simulink model "FDIBenchMark_66"  (Simulink 7.0)
settings: Solver=ode45  StartTime=0.0  StopTime=4400  FixedStep=Ts  RelTol=1e-12
InitFcn:
  | FDIBenchMarkData
values from neighbouring files (symbols this model uses):
  a = 2.2    [FDIBenchMarkData.m]
  Addt = [-(B_dt+B_r)/J_r B_dt/N_g/J_r -K_dt/J_r; eta_dt*B_dt/N_g/J_g -(eta_dt*B_dt/N_g^2+B_g)/J_g eta_dt*K_dt/N_g/J_g; 1 -1/N_g 0]    [FDIBenchMarkData.m]
  Addt2 = [-(B_dt+B_r)/J_r B_dt/N_g/J_r -K_dt/J_r; eta_dt2*B_dt/N_g/J_g -(eta_dt2*B_dt/N_g^2+B_g)/J_g eta_dt2*K_dt/N_g/J_g; 1 -1/N_g 0]    [FDIBenchMarkData.m]
  alpha = 0.1    [FDIBenchMarkData.m]
  alpha_gc = 50    [FDIBenchMarkData.m]
  Bddt = [1/J_r 0; 0 -1/J_g;0 0]    [FDIBenchMarkData.m]
  Bddt2 = [1/J_r 0; 0 -1/J_g;0 0]    [FDIBenchMarkData.m]
  Cddt = [1 0 0;0 1 0]    [FDIBenchMarkData.m]
  Constant_Beta_1_m1 = 5    [FDIBenchMarkData.m]
  Constant_Beta_3_m1 = 10    [FDIBenchMarkData.m]
  Constant_Omega_r_m1 = 1.4    [FDIBenchMarkData.m]
  Constant_tau_gc = 100    [FDIBenchMarkData.m]
  eta_gc = 0.98    [FDIBenchMarkData.m]
  Gain_Beta_2_m2 = 1.2    [FDIBenchMarkData.m]
  Gain_Omega_r_m2 = 1.1    [FDIBenchMarkData.m]
  H = 87    [FDIBenchMarkData.m]
  k = 4.7    [FDIBenchMarkData.m]
  K_i = 1    [FDIBenchMarkData.m]
  K_opt = .5* rho* pi*R^2*eta_dt*R^3*0.4554/(N_g*8)^3    (= 1.21708013189)    [FDIBenchMarkData.m]
  K_p = 4    [FDIBenchMarkData.m]
  L = acker(A', C', vpe)'    [FDIBenchMarkData.m]
  m = 1+alpha*(alpha-1)*R^2/(8*H^2)    (= 0.995085835315)    [FDIBenchMarkData.m]
  m_Beta = 0    [FDIBenchMarkData.m]
  m_omega_g = 0    [FDIBenchMarkData.m]
  m_omega_r = 0    [FDIBenchMarkData.m]
  m_P_g = 0    [FDIBenchMarkData.m]
  m_tau_g = 0    [FDIBenchMarkData.m]
  m_vw = 1.5    [FDIBenchMarkData.m]
  Omega_delta = 15    [FDIBenchMarkData.m]
  omega_n = 11.11    [FDIBenchMarkData.m]
  Omega_nom = 162    [FDIBenchMarkData.m]
  P_r = 4.8e6    (= 4800000)    [FDIBenchMarkData.m]
  R = 57.5    [FDIBenchMarkData.m]
  r = D_rotor/2    (= 57.5)    [FDIBenchMarkData.m]
  r0 = 1.5    [FDIBenchMarkData.m]
  rho = 1.225    [FDIBenchMarkData.m]
  seed = ceil(seed)    [FDIBenchMarkData.m]
  sigma_Beta = 0.2    [FDIBenchMarkData.m]
  sigma_omega_g = 0.05    [FDIBenchMarkData.m]
  sigma_omega_r = 0.004*2*pi    (= 0.0251327412287)    [FDIBenchMarkData.m]
  sigma_P_g = 1e3    (= 1000)    [FDIBenchMarkData.m]
  sigma_tau_g = 90    [FDIBenchMarkData.m]
  sigma_vm = 0.5    [FDIBenchMarkData.m]
  T_sample = 0.05    [FDIBenchMarkData.m]
  Ts = 1/100    (= 0.01)    [FDIBenchMarkData.m]
  turb_int = Turbulence_intensity    (= 12)    [FDIBenchMarkData.m]
  turbulence_seeds = [seed1 seed2]    [FDIBenchMarkData.m]
  xi = 0.6    [FDIBenchMarkData.m]
undefined symbols (not defined in the file or in its folder): Apb, Apb1, Apb2, Bpb, Bpb1, Bpb2, Cpb, Cpb1, Cpb2, Cq, DiscIntNeverNeededParam, u0
(part 1 of 2)
settings Model: Creator=peodg  LastModifiedBy=peodg
settings SolverCC: MaxConsecutiveZCs=1e6
settings HardwareCC: TargetHWDeviceType=32-bit Generic
settings GRTTargetCC: TargetFcnLib=ansi_tfl_tmw.mat

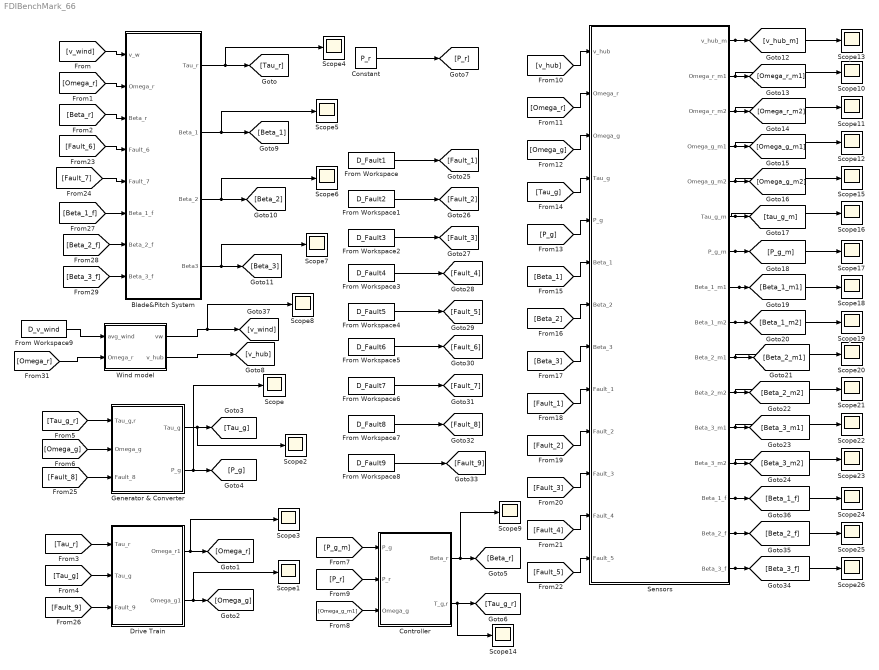
== system FDIBenchMark_66 ==
  Blade&Pitch System : Subsystem
  Constant : Constant  Value=P_r  OutDataType=sfix(16)  OutScaling=2^0
  Controller : Subsystem
  Drive Train : Subsystem
  From Workspace : FromWorkspace  VariableName=D_Fault1  SampleTime=Ts
  From Workspace1 : FromWorkspace  VariableName=D_Fault2  SampleTime=Ts
  From Workspace2 : FromWorkspace  VariableName=D_Fault3  SampleTime=Ts
  From Workspace3 : FromWorkspace  VariableName=D_Fault4  SampleTime=Ts
  From Workspace4 : FromWorkspace  VariableName=D_Fault5  SampleTime=Ts
  From Workspace5 : FromWorkspace  VariableName=D_Fault6  SampleTime=Ts
  From Workspace6 : FromWorkspace  VariableName=D_Fault7  SampleTime=Ts
  From Workspace7 : FromWorkspace  VariableName=D_Fault8  SampleTime=Ts
  From Workspace8 : FromWorkspace  VariableName=D_Fault9  SampleTime=Ts
  From Workspace9 : FromWorkspace  VariableName=D_v_wind
  Generator & Converter : Subsystem
  Scope{,1..26} (27 alike) : Scope
      Scope settings: YMin=1e+006  YMax=5.25e+006  SaveName=P_g  DataFormat=Array  SampleInput=on  SampleTime=Ts
      Scope1 settings: YMin=64  YMax=66.25  SaveName=Oemga_g1  DataFormat=Array  SampleInput=on  SampleTime=Ts
      Scope10 settings: YMin=1.1  YMax=2.4  SaveName=Omega_r_m1  DataFormat=Array  SampleInput=on  SampleTime=Ts
      Scope11 settings: YMin=-1  YMax=1  SaveName=Omega_r_m2  DataFormat=Array  SampleInput=on  SampleTime=Ts
      Scope12 settings: YMin=-1  YMax=1  SaveName=Omega_g_m1  DataFormat=Array  SampleInput=on  SampleTime=Ts
      Scope13 settings: YMin=-1  YMax=1  SaveName=v_hub_m  DataFormat=Array  SampleInput=on  SampleTime=Ts
      Scope14 settings: YMin=-2.5  YMax=20  SaveName=T_g_r  DataFormat=Array  SampleInput=on  SampleTime=Ts
      Scope15 settings: YMin=-1  YMax=1  SaveName=Omega_g_m2  DataFormat=Array  SampleInput=on  SampleTime=Ts
      Scope16 settings: YMin=-1  YMax=1  SaveName=Tau_g_m  DataFormat=Array  SampleInput=on  SampleTime=Ts
      Scope17 settings: YMin=-1  YMax=1  SaveName=P_g_m  DataFormat=Array  SampleInput=on  SampleTime=Ts
      Scope18 settings: YMin=-1  YMax=1  SaveName=Beta_1_m1  DataFormat=Array  SampleInput=on  SampleTime=Ts
      Scope19 settings: YMin=-1  YMax=1  SaveName=Beta_1_m2  DataFormat=Array  SampleInput=on  SampleTime=Ts
      Scope2 settings: YMin=29400  YMax=29875  SaveName=Tau_g  DataFormat=Array  SampleInput=on  SampleTime=Ts
      Scope20 settings: YMin=-1  YMax=1  SaveName=Beta_2_m1  DataFormat=Array  SampleInput=on  SampleTime=Ts
      Scope21 settings: YMin=-1  YMax=1  SaveName=Beta_2_m2  DataFormat=Array  SampleInput=on  SampleTime=Ts
      Scope22 settings: YMin=-1  YMax=1  SaveName=Beta_3_m1  DataFormat=Array  SampleInput=on  SampleTime=Ts
      Scope23 settings: YMin=-1  YMax=1  SaveName=Beta_3_m2  DataFormat=Array  SampleInput=on  SampleTime=Ts
      Scope24 settings: YMin=-1  YMax=1  SaveName=Beta_1_f  DataFormat=Array  SampleInput=on  SampleTime=Ts
      Scope25 settings: YMin=-1  YMax=1  SaveName=Beta_2_f  DataFormat=Array  SampleInput=on  SampleTime=Ts
      Scope26 settings: YMin=-1  YMax=1  SaveName=Beta_3_f  DataFormat=Array  SampleInput=on  SampleTime=Ts
      Scope3 settings: YMin=0.62  YMax=0.69  SaveName=Omega_r1  DataFormat=Array  SampleInput=on  SampleTime=Ts
      Scope4 settings: YMin=-1e+006  YMax=6e+006  SaveName=Tau_r  DataFormat=Array  SampleInput=on  SampleTime=Ts
      Scope5 settings: YMin=-3  YMax=8  SaveName=Beta1  DataFormat=Array  SampleInput=on  SampleTime=Ts
      Scope6 settings: YMin=-0.3  YMax=0.3  SaveName=Beta  DataFormat=Array  SampleInput=on  SampleTime=Ts
      Scope7 settings: YMin=-0.25  YMax=0.35  SaveName=Beta3  DataFormat=Array  SampleInput=on  SampleTime=Ts
      Scope8 settings: YMin=3  YMax=18  SaveName=Vw  DataFormat=Array  SampleInput=on  SampleTime=Ts
      Scope9 settings: YMin=-2.5  YMax=20  SaveName=Beta_r  DataFormat=Array  SampleInput=on  SampleTime=Ts
  Sensors : Subsystem
  Wind model : Subsystem
  wires:
  [v_wind] -> Blade&Pitch System/1(v_w)
  [Omega_r] -> Blade&Pitch System/2(Omega_r)
  [Beta_r] -> Blade&Pitch System/3(Beta_r)
  [Tau_r] -> Drive Train/1(Tau_r)
  [Tau_g] -> Drive Train/2(Tau_g)
  Drive Train/1(Omega_r1) -> [Omega_r], Scope3/1
  [Tau_g_r] -> Generator & Converter/1(Tau_g,r)
  [Omega_g] -> Generator & Converter/2(Omega_g)
  Generator & Converter/1(Tau_g) -> [Tau_g], Scope2/1
  Generator & Converter/2(P_g) -> [P_g], Scope/1
  [P_g_m] -> Controller/1(P_g)
  [Omega_g_m1] -> Controller/3(Omega_g)
  Controller/1(Beta_r) -> [Beta_r], Scope9/1
  Controller/2(T_g,r) -> [Tau_g_r], Scope14/1
  [P_r] -> Controller/2(P_r)
  Constant/1 -> [P_r]
  Sensors/1(v_hub_m) -> [v_hub_m], Scope13/1
  Sensors/2(Omega_r_m1) -> [Omega_r_m1], Scope10/1
  Sensors/3(Omega_r_m2) -> [Omega_r_m2], Scope11/1
  Sensors/4(Omega_g_m1) -> [Omega_g_m1], Scope12/1
  Sensors/5(Omega_g_m2) -> [Omega_g_m2], Scope15/1
  Sensors/6(Tau_g_m) -> [tau_g_m], Scope16/1
  Sensors/7(P_g_m) -> [P_g_m], Scope17/1
  Sensors/8(Beta_1_m1) -> [Beta_1_m1], Scope18/1
  Sensors/9(Beta_1_m2) -> [Beta_1_m2], Scope19/1
  Sensors/10(Beta_2_m1) -> [Beta_2_m1], Scope20/1
  Sensors/11(Beta_2_m2) -> [Beta_2_m2], Scope21/1
  Sensors/12(Beta_3_m1) -> [Beta_3_m1], Scope22/1
  Sensors/13(Beta_3_m2) -> [Beta_3_m2], Scope23/1
  [v_hub] -> Sensors/1(v_hub)
  [Omega_r] -> Sensors/2(Omega_r)
  [Omega_g] -> Sensors/3(Omega_g)
  [Tau_g] -> Sensors/4(Tau_g)
  [P_g] -> Sensors/5(P_g)
  [Beta_1] -> Sensors/6(Beta_1)
  [Beta_2] -> Sensors/7(Beta_2)
  [Beta_3] -> Sensors/8(Beta_3)
  [Fault_1] -> Sensors/9(Fault_1)
  [Fault_2] -> Sensors/10(Fault_2)
  [Fault_3] -> Sensors/11(Fault_3)
  [Fault_4] -> Sensors/12(Fault_4)
  [Fault_5] -> Sensors/13(Fault_5)
  [Fault_6] -> Blade&Pitch System/4(Fault_6)
  [Fault_7] -> Blade&Pitch System/5(Fault_7)
  [Fault_8] -> Generator & Converter/3(Fault_8)
  [Fault_9] -> Drive Train/3(Fault_9)
  From Workspace8/1 -> [Fault_9]
  From Workspace7/1 -> [Fault_8]
  From Workspace6/1 -> [Fault_7]
  From Workspace5/1 -> [Fault_6]
  From Workspace4/1 -> [Fault_5]
  From Workspace3/1 -> [Fault_4]
  From Workspace2/1 -> [Fault_3]
  From Workspace1/1 -> [Fault_2]
  From Workspace/1 -> [Fault_1]
  Drive Train/2(Omega_g1) -> [Omega_g], Scope1/1
  Sensors/16(Beta_3_f) -> [Beta_3_f], Scope26/1
  Sensors/15(Beta_2_f) -> [Beta_2_f], Scope25/1
  Sensors/14(Beta_1_f) -> [Beta_1_f], Scope24/1
  [Beta_1_f] -> Blade&Pitch System/6(Beta_1_f)
  [Beta_2_f] -> Blade&Pitch System/7(Beta_2_f)
  [Beta_3_f] -> Blade&Pitch System/8(Beta_3_f)
  Blade&Pitch System/4(Beta3) -> [Beta_3], Scope7/1
  Blade&Pitch System/3(Beta_2) -> [Beta_2], Scope6/1
  Blade&Pitch System/2(Beta_1) -> [Beta_1], Scope5/1
  Blade&Pitch System/1(Tau_r) -> [Tau_r], Scope4/1
  Wind model/1(vw) -> [v_wind], Scope8/1
  Wind model/2(v_hub) -> [v_hub]
  [Omega_r] -> Wind model/2(Omega_r)
  From Workspace9/1 -> Wind model/1(avg_wind)

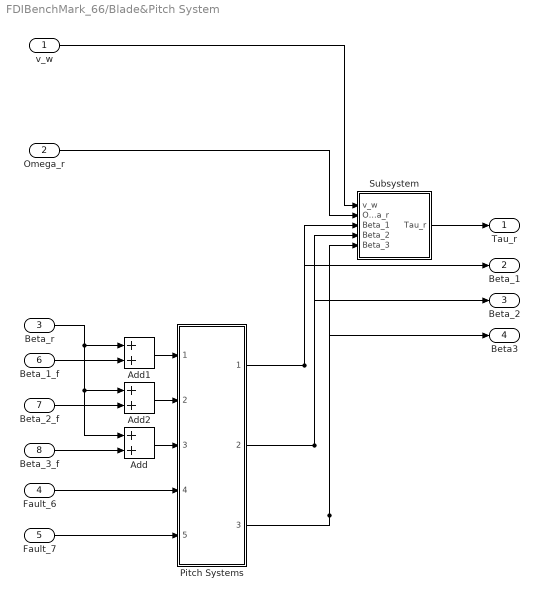
== system FDIBenchMark_66/Blade&Pitch System ==
  v_w : Inport  OutDataType=sfix(16)  OutScaling=2^0
  Omega_r : Inport  Port=2  OutDataType=sfix(16)  OutScaling=2^0
  Beta_r : Inport  Port=3  OutDataType=sfix(16)  OutScaling=2^0
  Fault_6 : Inport  Port=4  OutDataType=sfix(16)  OutScaling=2^0
  Fault_7 : Inport  Port=5  OutDataType=sfix(16)  OutScaling=2^0
  Beta_1_f : Inport  Port=6  OutDataType=sfix(16)  OutScaling=2^0
  Beta_2_f : Inport  Port=7  OutDataType=sfix(16)  OutScaling=2^0
  Beta_3_f : Inport  Port=8  OutDataType=sfix(16)  OutScaling=2^0
  Add : Sum  OutDataType=sfix(16)  OutScaling=2^-10
  Add1 : Sum  OutDataType=sfix(16)  OutScaling=2^-10
  Add2 : Sum  OutDataType=sfix(16)  OutScaling=2^-10
  Pitch Systems : Subsystem
  Subsystem : Subsystem
  Tau_r : Outport  OutDataType=sfix(16)  OutScaling=2^0
  Beta_1 : Outport  Port=2  OutDataType=sfix(16)  OutScaling=2^0
  Beta_2 : Outport  Port=3  OutDataType=sfix(16)  OutScaling=2^0
  Beta3 : Outport  Port=4  OutDataType=sfix(16)  OutScaling=2^0
  wires:
  Pitch Systems/1(Beta_1) -> Subsystem/3(Beta_1), Beta_1/1
  Pitch Systems/2(Beta_2) -> Subsystem/4(Beta_2), Beta_2/1
  Pitch Systems/3(Beta_3) -> Subsystem/5(Beta_3), Beta3/1
  Subsystem/1(Tau_r) -> Tau_r/1
  v_w/1 -> Subsystem/1(v_w)
  Omega_r/1 -> Subsystem/2(Omega_r)
  Fault_6/1 -> Pitch Systems/4(Fault_6)
  Fault_7/1 -> Pitch Systems/5(Fault_7)
  Add/1 -> Pitch Systems/3(Beta_r3)
  Add1/1 -> Pitch Systems/1(Beta_r1)
  Add2/1 -> Pitch Systems/2(Beta_r2)
  Beta_3_f/1 -> Add/2
  Beta_2_f/1 -> Add2/2
  Beta_1_f/1 -> Add1/2
  Beta_r/1 -> Add1/1, Add2/1, Add/1

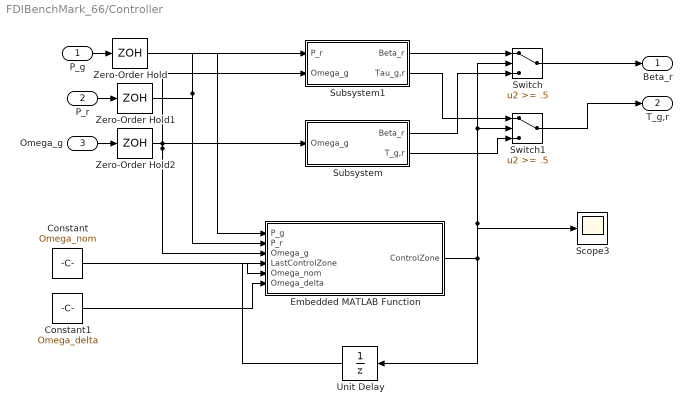
== system FDIBenchMark_66/Controller ==
  P_g : Inport  OutDataType=sfix(16)  OutScaling=2^0
  P_r : Inport  Port=2  OutDataType=sfix(16)  OutScaling=2^0
  Omega_g : Inport  Port=3  OutDataType=sfix(16)  OutScaling=2^0
  Constant : Constant  Value=Omega_nom  OutDataType=sfix(16)  OutScaling=2^0
  Constant1 : Constant  Value=Omega_delta  OutDataType=sfix(16)  OutScaling=2^0
  Embedded MATLAB Function : Stateflow chart
      settings: PermitHierarchicalResolution=ParametersOnly
  Scope3 : Scope
      settings: YMin=0.62  YMax=0.69  SaveName=Omega_r  DataFormat=Array  SampleInput=on  SampleTime=Ts
  Subsystem : Subsystem
  Subsystem1 : Subsystem
  Switch : Switch  Threshold=.5
  Switch1 : Switch  Threshold=.5
  Unit Delay : UnitDelay  Orientation=left  SampleTime=Ts
  Zero-Order Hold : ZeroOrderHold  SampleTime=Ts
  Zero-Order Hold1 : ZeroOrderHold  SampleTime=Ts
  Zero-Order Hold2 : ZeroOrderHold  SampleTime=Ts
  Beta_r : Outport  OutDataType=sfix(16)  OutScaling=2^0
  T_g,r : Outport  Port=2  OutDataType=sfix(16)  OutScaling=2^0
  wires:
  Embedded MATLAB Function/1(ControlZone) -> Unit Delay/1, Switch/2, Switch1/2, Scope3/1
  Unit Delay/1 -> Embedded MATLAB Function/4(LastControlZone)
  P_g/1 -> Zero-Order Hold/1
  P_r/1 -> Zero-Order Hold1/1
  Omega_g/1 -> Zero-Order Hold2/1
  Switch/1 -> Beta_r/1
  Switch1/1 -> T_g,r/1
  Subsystem1/1(Beta_r) -> Switch/1
  Subsystem/1(Beta_r) -> Switch/3
  Subsystem1/2(Tau_g,r) -> Switch1/1
  Subsystem/2(T_g,r) -> Switch1/3
  Constant/1 -> Embedded MATLAB Function/5(Omega_nom)
  Constant1/1 -> Embedded MATLAB Function/6(Omega_delta)
  Zero-Order Hold/1 -> Embedded MATLAB Function/1(P_g)
  Zero-Order Hold1/1 -> Embedded MATLAB Function/2(P_r), Subsystem1/1(P_r)
  Zero-Order Hold2/1 -> Embedded MATLAB Function/3(Omega_g), Subsystem1/2(Omega_g), Subsystem/1(Omega_g)

== system FDIBenchMark_66/Drive Train ==
  Tau_r : Inport  OutDataType=sfix(16)  OutScaling=2^0
  Tau_g : Inport  Port=2  OutDataType=sfix(16)  OutScaling=2^0
  Fault_9 : Inport  Port=3  OutDataType=sfix(16)  OutScaling=2^0
  Add : Sum  OutDataType=sfix(16)  OutScaling=2^-10
  Demux1 : Demux  Outputs=2
  Gain : Gain  Orientation=left  Gain=Addt  Multiplication=Matrix(K*u)  ParameterDataType=sfix(16)  ParameterScaling=2^0  OutDataType=sfix(16)  OutScaling=2^0
  Gain1 : Gain  Gain=Bddt  Multiplication=Matrix(K*u)  ParameterDataType=sfix(16)  ParameterScaling=2^0  OutDataType=sfix(16)  OutScaling=2^0
  Gain2 : Gain  Gain=Cddt  Multiplication=Matrix(K*u)  ParameterDataType=sfix(16)  ParameterScaling=2^0  OutDataType=sfix(16)  OutScaling=2^0
  Gain3 : Gain  Orientation=left  Gain=Addt2  Multiplication=Matrix(K*u)  ParameterDataType=sfix(16)  ParameterScaling=2^0  OutDataType=sfix(16)  OutScaling=2^0
  Gain4 : Gain  Gain=Bddt2  Multiplication=Matrix(K*u)  ParameterDataType=sfix(16)  ParameterScaling=2^0  OutDataType=sfix(16)  OutScaling=2^0
  Integrator : Integrator  InitialCondition=[1 100 0]
  Mux : Mux  Inputs=2
  Switch1 : Switch  Threshold=0.5
  Switch2 : Switch  Orientation=left  Threshold=0.5
  Omega_r1 : Outport  OutDataType=sfix(16)  OutScaling=2^0
  Omega_g1 : Outport  Port=2  OutDataType=sfix(16)  OutScaling=2^0
  wires:
  Tau_r/1 -> Mux/1
  Tau_g/1 -> Mux/2
  Integrator/1 -> Gain2/1, Gain/1, Gain3/1
  Add/1 -> Integrator/1
  Switch1/1 -> Add/1
  Gain1/1 -> Switch1/1
  Gain4/1 -> Switch1/3
  Gain/1 -> Switch2/1
  Gain3/1 -> Switch2/3
  Switch2/1 -> Add/2
  Demux1/1 -> Omega_r1/1
  Demux1/2 -> Omega_g1/1
  Gain2/1 -> Demux1/1
  Fault_9/1 -> Switch1/2, Switch2/2
  Mux/1 -> Gain1/1, Gain4/1

== system FDIBenchMark_66/Generator & Converter ==
  Tau_g,r : Inport  OutDataType=sfix(16)  OutScaling=2^0
  Omega_g : Inport  Port=2  OutDataType=sfix(16)  OutScaling=2^0
  Fault_8 : Inport  Port=3  OutDataType=sfix(16)  OutScaling=2^0
  Bias : Bias  Bias=Constant_tau_gc
  Divide : Product  Inputs=**  OutDataType=sfix(16)  OutScaling=2^-10
  Gain : Gain  Gain=eta_gc  ParameterDataType=sfix(16)  ParameterScaling=2^0  OutDataType=sfix(16)  OutScaling=2^0
  Switch : Switch  Threshold=0.5
  Transfer Fcn : TransferFcn  Numerator=[alpha_gc]  Denominator=[1 alpha_gc]
  Tau_g : Outport  OutDataType=sfix(16)  OutScaling=2^0
  P_g : Outport  Port=2  OutDataType=sfix(16)  OutScaling=2^0
  wires:
  Tau_g,r/1 -> Transfer Fcn/1
  Gain/1 -> P_g/1
  Divide/1 -> Gain/1
  Omega_g/1 -> Divide/2
  Transfer Fcn/1 -> Bias/1, Switch/1
  Fault_8/1 -> Switch/2
  Switch/1 -> Divide/1, Tau_g/1
  Bias/1 -> Switch/3

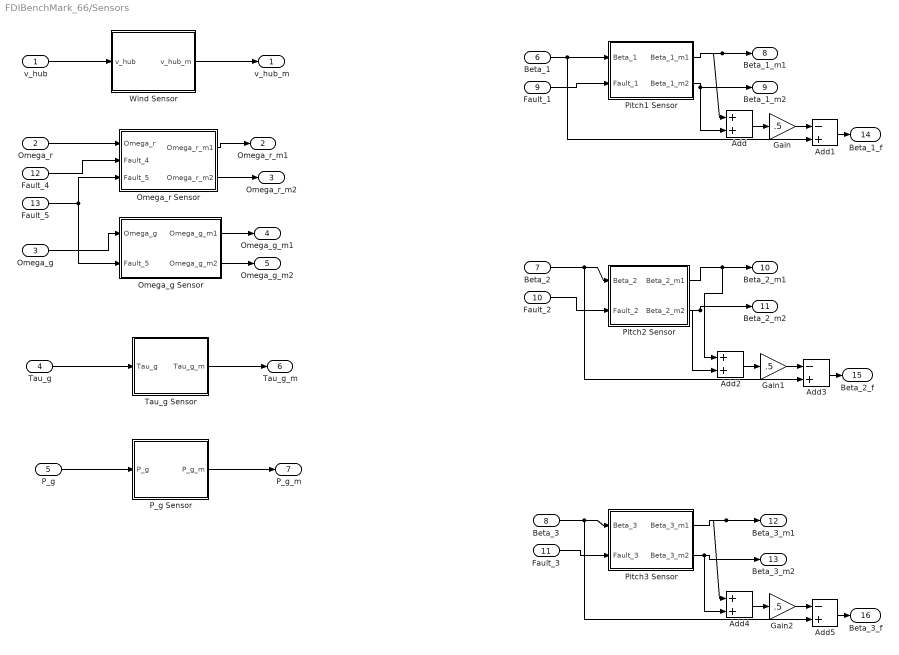
== system FDIBenchMark_66/Sensors ==
  v_hub : Inport  OutDataType=sfix(16)  OutScaling=2^0
  Omega_r : Inport  Port=2  OutDataType=sfix(16)  OutScaling=2^0
  Omega_g : Inport  Port=3  OutDataType=sfix(16)  OutScaling=2^0
  Tau_g : Inport  Port=4  OutDataType=sfix(16)  OutScaling=2^0
  P_g : Inport  Port=5  OutDataType=sfix(16)  OutScaling=2^0
  Beta_1 : Inport  Port=6  OutDataType=sfix(16)  OutScaling=2^0
  Beta_2 : Inport  Port=7  OutDataType=sfix(16)  OutScaling=2^0
  Beta_3 : Inport  Port=8  OutDataType=sfix(16)  OutScaling=2^0
  Fault_1 : Inport  Port=9  OutDataType=sfix(16)  OutScaling=2^0
  Fault_2 : Inport  Port=10  OutDataType=sfix(16)  OutScaling=2^0
  Fault_3 : Inport  Port=11  OutDataType=sfix(16)  OutScaling=2^0
  Fault_4 : Inport  Port=12  OutDataType=sfix(16)  OutScaling=2^0
  Fault_5 : Inport  Port=13  OutDataType=sfix(16)  OutScaling=2^0
  Add : Sum  OutDataType=sfix(16)  OutScaling=2^-10
  Add1 : Sum  Inputs=-+  OutDataType=sfix(16)  OutScaling=2^-10
  Add2 : Sum  OutDataType=sfix(16)  OutScaling=2^-10
  Add3 : Sum  Inputs=-+  OutDataType=sfix(16)  OutScaling=2^-10
  Add4 : Sum  OutDataType=sfix(16)  OutScaling=2^-10
  Add5 : Sum  Inputs=-+  OutDataType=sfix(16)  OutScaling=2^-10
  Gain : Gain  Gain=.5  ParameterDataType=sfix(16)  ParameterScaling=2^0  OutDataType=sfix(16)  OutScaling=2^0
  Gain1 : Gain  Gain=.5  ParameterDataType=sfix(16)  ParameterScaling=2^0  OutDataType=sfix(16)  OutScaling=2^0
  Gain2 : Gain  Gain=.5  ParameterDataType=sfix(16)  ParameterScaling=2^0  OutDataType=sfix(16)  OutScaling=2^0
  Omega_g Sensor : Subsystem
  Omega_r Sensor : Subsystem
  P_g Sensor : Subsystem
  Pitch1 Sensor : Subsystem
  Pitch2 Sensor : Subsystem
  Pitch3 Sensor : Subsystem
  Tau_g Sensor : Subsystem
  Wind Sensor : Subsystem
  v_hub_m : Outport  OutDataType=sfix(16)  OutScaling=2^0
  Omega_r_m1 : Outport  Port=2  OutDataType=sfix(16)  OutScaling=2^0
  Omega_r_m2 : Outport  Port=3  OutDataType=sfix(16)  OutScaling=2^0
  Omega_g_m1 : Outport  Port=4  OutDataType=sfix(16)  OutScaling=2^0
  Omega_g_m2 : Outport  Port=5  OutDataType=sfix(16)  OutScaling=2^0
  Tau_g_m : Outport  Port=6  OutDataType=sfix(16)  OutScaling=2^0
  P_g_m : Outport  Port=7  OutDataType=sfix(16)  OutScaling=2^0
  Beta_1_m1 : Outport  Port=8  OutDataType=sfix(16)  OutScaling=2^0
  Beta_1_m2 : Outport  Port=9  OutDataType=sfix(16)  OutScaling=2^0
  Beta_2_m1 : Outport  Port=10  OutDataType=sfix(16)  OutScaling=2^0
  Beta_2_m2 : Outport  Port=11  OutDataType=sfix(16)  OutScaling=2^0
  Beta_3_m1 : Outport  Port=12  OutDataType=sfix(16)  OutScaling=2^0
  Beta_3_m2 : Outport  Port=13  OutDataType=sfix(16)  OutScaling=2^0
  Beta_1_f : Outport  Port=14  OutDataType=sfix(16)  OutScaling=2^0
  Beta_2_f : Outport  Port=15  OutDataType=sfix(16)  OutScaling=2^0
  Beta_3_f : Outport  Port=16  OutDataType=sfix(16)  OutScaling=2^0
  wires:
  Wind Sensor/1(v_hub_m) -> v_hub_m/1
  v_hub/1 -> Wind Sensor/1(v_hub)
  Omega_r/1 -> Omega_r Sensor/1(Omega_r)
  Omega_r Sensor/1(Omega_r_m1) -> Omega_r_m1/1
  Omega_r Sensor/2(Omega_r_m2) -> Omega_r_m2/1
  Omega_g/1 -> Omega_g Sensor/1(Omega_g)
  Omega_g Sensor/1(Omega_g_m1) -> Omega_g_m1/1
  Omega_g Sensor/2(Omega_g_m2) -> Omega_g_m2/1
  Tau_g/1 -> Tau_g Sensor/1(Tau_g)
  Tau_g Sensor/1(Tau_g_m) -> Tau_g_m/1
  P_g/1 -> P_g Sensor/1(P_g)
  P_g Sensor/1(P_g_m) -> P_g_m/1
  Beta_1/1 -> Pitch1 Sensor/1(Beta_1), Add1/2
  Pitch1 Sensor/1(Beta_1_m1) -> Beta_1_m1/1, Add/1
  Pitch1 Sensor/2(Beta_1_m2) -> Beta_1_m2/1, Add/2
  Beta_2/1 -> Pitch2 Sensor/1(Beta_2), Add3/2
  Pitch2 Sensor/1(Beta_2_m1) -> Beta_2_m1/1, Add2/1
  Pitch2 Sensor/2(Beta_2_m2) -> Beta_2_m2/1, Add2/2
  Beta_3/1 -> Pitch3 Sensor/1(Beta_3), Add5/2
  Pitch3 Sensor/1(Beta_3_m1) -> Beta_3_m1/1, Add4/1
  Pitch3 Sensor/2(Beta_3_m2) -> Beta_3_m2/1, Add4/2
  Fault_1/1 -> Pitch1 Sensor/2(Fault_1)
  Fault_2/1 -> Pitch2 Sensor/2(Fault_2)
  Fault_3/1 -> Pitch3 Sensor/2(Fault_3)
  Fault_4/1 -> Omega_r Sensor/2(Fault_4)
  Fault_5/1 -> Omega_r Sensor/3(Fault_5), Omega_g Sensor/2(Fault_5)
  Add/1 -> Gain/1
  Gain/1 -> Add1/1
  Add1/1 -> Beta_1_f/1
  Add2/1 -> Gain1/1
  Gain1/1 -> Add3/1
  Add3/1 -> Beta_2_f/1
  Add4/1 -> Gain2/1
  Gain2/1 -> Add5/1
  Add5/1 -> Beta_3_f/1

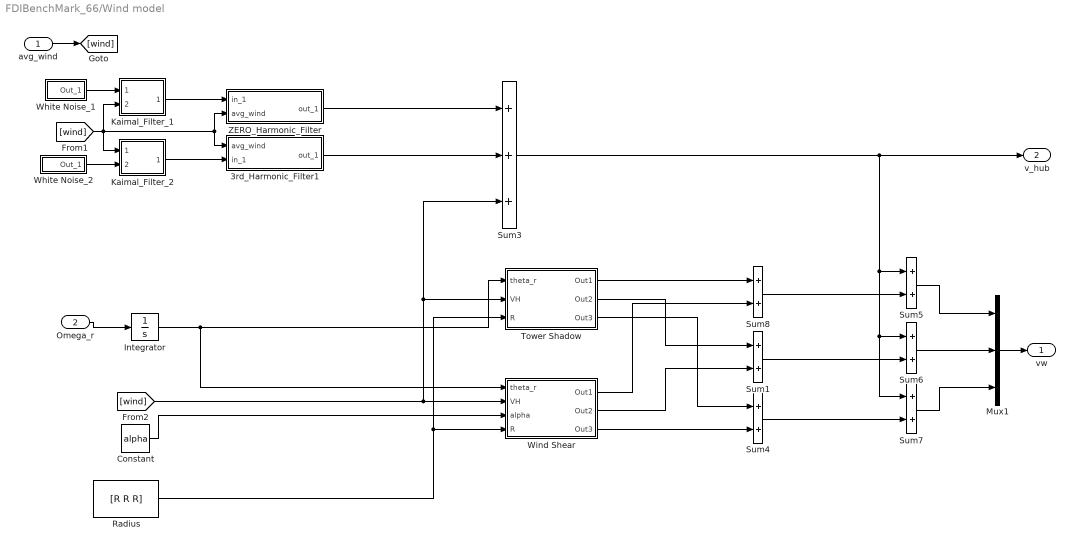
== system FDIBenchMark_66/Wind model ==
  avg_wind : Inport  OutDataType=sfix(16)  OutScaling=2^0
  Omega_r : Inport  Port=2  OutDataType=sfix(16)  OutScaling=2^0
  3rd_Harmonic_Filter1 : Subsystem
  Constant : Constant  Value=alpha  OutDataType=sfix(16)  OutScaling=2^0
  Integrator : Integrator
  Kaimal_Filter_1 : Subsystem
  Kaimal_Filter_2 : Subsystem
  Mux1 : Mux  Inputs=3
  Radius : Constant  Value=[R R R]  OutDataType=sfix(16)  OutScaling=2^0
  Sum{1,4..8} (6 alike) : Sum  OutDataType=sfix(16)  OutScaling=2^0  SaturateOnIntegerOverflow=on  InputSameDT=on
  Sum3 : Sum  Inputs=+++  OutDataType=sfix(16)  OutScaling=2^0  SaturateOnIntegerOverflow=on  InputSameDT=on
  Tower Shadow : Subsystem
  White Noise_1 : Subsystem  mask(Continuous White Noise.){Cov=[1], Ts=T_sample, seed=turbulence_seeds(1)}
      mask prompts: Cov "Noise Power:"; Ts "Sample Time:"
      mask help:
      | White noise for continuous (s-domain) systems.
      | Band-limited using zero-order-hold.
      mask init:
      | r = rand(1,12); r2 = [r(1),r;r,r(12)]; t =[1:13;1:13];
      mask Help: Implemented using white noise into Zero-Order Hold block. The seed and power can be vectors of the same length to produce a vector of white noise sources. For faster simulation, set sample time to the highest value possible but in accordance with the fastest dynamics of system.
      mask Display: plot(t(:),r2(:))
  White Noise_2 : Subsystem  mask(Continuous White Noise.){@1=[1], @2=T_sample, @3=turbulence_seeds(2)}
      mask prompts: @1 "Noise Power:"; @2 "Sample Time:"; @3 "Seed"
      mask help:
      | White noise for continuous (s-domain) systems.
      | Band-limited using zero-order-hold.
      mask init:
      | Cov = @1; Ts = @2; seed = @3; r = rand(1,12); r2 = [r(1),r;r,r(12)]; t =[1:13;1:13];
      mask Help: Implemented using white noise into Zero-Order Hold block. The seed and power can be vectors of the same length to produce a vector of white noise sources. For faster simulation, set sample time to the highest value possible but in accordance with the fastest dynamics of system.
      mask Display: plot(t(:),r2(:))
  Wind Shear : Subsystem
  ZERO_Harmonic_Filter : Subsystem
  vw : Outport  OutDataType=sfix(16)  OutScaling=2^0  InitialOutput=[u0]
  v_hub : Outport  Port=2  OutDataType=sfix(16)  OutScaling=2^0  InitialOutput=[u0]
  wires:
  [wind] -> 3rd_Harmonic_Filter1/1(avg_wind), ZERO_Harmonic_Filter/2(avg_wind), Kaimal_Filter_2/1(avg_wind), Kaimal_Filter_1/2(avg_wind)
  avg_wind/1 -> [wind]
  White Noise_2/1(Out_1) -> Kaimal_Filter_2/2(in_1)
  Kaimal_Filter_2/1(out_1) -> 3rd_Harmonic_Filter1/2(in_1)
  Kaimal_Filter_1/1(out_1) -> ZERO_Harmonic_Filter/1(in_1)
  White Noise_1/1(Out_1) -> Kaimal_Filter_1/1(in_1)
  [wind] -> Wind Shear/2(VH), Sum3/3, Tower Shadow/2(VH)
  Constant/1 -> Wind Shear/3(alpha)
  Radius/1 -> Wind Shear/4(R), Tower Shadow/3(R)
  Tower Shadow/1(Out1) -> Sum8/1
  Wind Shear/1(Out1) -> Sum8/2
  Tower Shadow/2(Out2) -> Sum1/1
  Wind Shear/2(Out2) -> Sum1/2
  Tower Shadow/3(Out3) -> Sum4/1
  Wind Shear/3(Out3) -> Sum4/2
  Sum8/1 -> Sum5/2
  Sum1/1 -> Sum6/2
  Sum4/1 -> Sum7/2
  Sum5/1 -> Mux1/1
  Sum6/1 -> Mux1/2
  Sum7/1 -> Mux1/3
  Mux1/1 -> vw/1
  Sum3/1 -> Sum6/1, Sum7/1, Sum5/1, v_hub/1
  3rd_Harmonic_Filter1/1(out_1) -> Sum3/2
  ZERO_Harmonic_Filter/1(out_1) -> Sum3/1
  Omega_r/1 -> Integrator/1
  Integrator/1 -> Tower Shadow/1(theta_r), Wind Shear/1(theta_r)

== system FDIBenchMark_66/Blade&Pitch System/Pitch Systems ==
  Beta_r1 : Inport
  Beta_r2 : Inport  Port=2
  Beta_r3 : Inport  Port=3
  Fault_6 : Inport  Port=4
  Fault_7 : Inport  Port=5
  PitchSystem 1 : Subsystem
  PitchSystem 2 : Subsystem
  PitchSystem 3 : Subsystem
  Beta_1 : Outport
  Beta_2 : Outport  Port=2
  Beta_3 : Outport  Port=3
  wires:
  PitchSystem 1/1(Beta_1) -> Beta_1/1
  PitchSystem 2/1(Beta_2) -> Beta_2/1
  PitchSystem 3/1(Beta_3) -> Beta_3/1
  Fault_7/1 -> PitchSystem 3/2(Fault_7)
  Fault_6/1 -> PitchSystem 2/2(Fault_6)
  Beta_r3/1 -> PitchSystem 3/1(Beta_r)
  Beta_r2/1 -> PitchSystem 2/1(Beta_r)
  Beta_r1/1 -> PitchSystem 1/1(Beta_r)

== system FDIBenchMark_66/Blade&Pitch System/Subsystem ==
  v_w : Inport
  Omega_r : Inport  Port=2
  Beta_1 : Inport  Port=3
  Beta_2 : Inport  Port=4
  Beta_3 : Inport  Port=5
  Add : Sum  Inputs=+++  OutDataType=sfix(16)  OutScaling=2^-10
  AeroDyn 1 : Subsystem
  AeroDyn 2 : Subsystem
  AeroDyn 3 : Subsystem
  Demux : Demux  Outputs=3
  Scope1 : Scope
      settings: YMin=0.5225  YMax=0.545  SaveName=ScopeData12
  Scope3 : Scope
      settings: YMin=5  YMax=7.75  SaveName=ScopeData11
  Tau_r : Outport
  wires:
  Omega_r/1 -> AeroDyn 1/2(Omega_r), AeroDyn 3/2(Omega_r), AeroDyn 2/2(Omega_r), Scope1/1
  AeroDyn 1/1(Tau_r1) -> Add/1
  AeroDyn 2/1(Tau_r2) -> Add/2
  AeroDyn 3/1(Tau_r3) -> Add/3
  Beta_1/1 -> AeroDyn 1/3(Beta_1)
  Add/1 -> Tau_r/1
  Beta_2/1 -> AeroDyn 2/3(Beta_2)
  Beta_3/1 -> AeroDyn 3/3(Beta_3)
  v_w/1 -> Demux/1, Scope3/1
  Demux/3 -> AeroDyn 3/1(v_w)
  Demux/2 -> AeroDyn 2/1(v_w)
  Demux/1 -> AeroDyn 1/1(v_w)

== system FDIBenchMark_66/Controller/Subsystem ==
  Omega_g : Inport  OutDataType=sfix(16)  OutScaling=2^0
  Constant : Constant  Value=0  OutDataType=sfix(16)  OutScaling=2^0
  Gain : Gain  Gain=K_opt  ParameterDataType=sfix(16)  ParameterScaling=2^0  OutDataType=sfix(16)  OutScaling=2^0
  Product : Product  OutDataType=sfix(16)  OutScaling=2^0  RndMeth=Zero
  Beta_r : Outport  OutDataType=sfix(16)  OutScaling=2^0
  T_g,r : Outport  Port=2  OutDataType=sfix(16)  OutScaling=2^0
  wires:
  Constant/1 -> Beta_r/1
  Omega_g/1 -> Product/2, Product/1
  Gain/1 -> T_g,r/1
  Product/1 -> Gain/1

== system FDIBenchMark_66/Controller/Subsystem1 ==
  P_r : Inport  OutDataType=sfix(16)  OutScaling=2^0
  Omega_g : Inport  Port=2  OutDataType=sfix(16)  OutScaling=2^0
  Add : Sum  OutDataType=sfix(16)  OutScaling=2^-10
  Bias : Bias  Bias=-Omega_nom
  Discrete-Time Integrator : DiscreteIntegrator  SampleTime=Ts  OutDataType=sfix(16)  OutScaling=2^0  LimitOutput=on  UpperSaturationLimit=90  LowerSaturationLimit=-2  ICPrevOutput=DiscIntNeverNeededParam  ICPrevScaledInput=DiscIntNeverNeededParam
  Divide : Product  Inputs=/*  OutDataType=sfix(16)  OutScaling=2^-10
  Gain : Gain  Gain=K_p  ParameterDataType=sfix(16)  ParameterScaling=2^0  OutDataType=sfix(16)  OutScaling=2^0
  Gain1 : Gain  Gain=K_i  ParameterDataType=sfix(16)  ParameterScaling=2^0  OutDataType=sfix(16)  OutScaling=2^0
  Gain2 : Gain  Gain=1/eta_gc  ParameterDataType=sfix(16)  ParameterScaling=2^0  OutDataType=sfix(16)  OutScaling=2^0
  Saturation : Saturate  UpperLimit=90  LowerLimit=-2
  Beta_r : Outport  OutDataType=sfix(16)  OutScaling=2^0
  Tau_g,r : Outport  Port=2  OutDataType=sfix(16)  OutScaling=2^0
  wires:
  Divide/1 -> Gain2/1
  P_r/1 -> Divide/2
  Omega_g/1 -> Divide/1, Bias/1
  Bias/1 -> Discrete-Time Integrator/1, Gain/1
  Discrete-Time Integrator/1 -> Gain1/1
  Gain1/1 -> Add/2
  Gain/1 -> Add/1
  Add/1 -> Saturation/1
  Saturation/1 -> Beta_r/1
  Gain2/1 -> Tau_g,r/1

== system FDIBenchMark_66/Sensors/Omega_g Sensor ==
  Omega_g : Inport
  Fault_5 : Inport  Port=2
  Add : Sum  OutDataType=sfix(16)  OutScaling=2^-10
  Add1 : Sum  OutDataType=sfix(16)  OutScaling=2^-10
  Gain : Gain  Gain=Gain_Omega_r_m2  ParameterDataType=sfix(16)  ParameterScaling=2^0  OutDataType=sfix(16)  OutScaling=2^0
  Random Number : RandomNumber  Mean=m_omega_g  Variance=sigma_omega_g  Seed=seed(4)  SampleTime=Ts
  Random Number1 : RandomNumber  Mean=m_omega_r  Variance=sigma_omega_r  Seed=seed(5)  SampleTime=Ts
  Switch1 : Switch  Threshold=0.5
  Omega_g_m1 : Outport
  Omega_g_m2 : Outport  Port=2
  wires:
  Random Number1/1 -> Add1/2
  Random Number/1 -> Add/1
  Omega_g/1 -> Add1/1, Add/2
  Add/1 -> Omega_g_m1/1
  Add1/1 -> Switch1/1, Gain/1
  Switch1/1 -> Omega_g_m2/1
  Fault_5/1 -> Switch1/2
  Gain/1 -> Switch1/3

== system FDIBenchMark_66/Sensors/Omega_r Sensor ==
  Omega_r : Inport
  Fault_4 : Inport  Port=2
  Fault_5 : Inport  Port=3
  Add : Sum  OutDataType=sfix(16)  OutScaling=2^-10
  Add1 : Sum  OutDataType=sfix(16)  OutScaling=2^-10
  Constant : Constant  Value=Constant_Omega_r_m1  OutDataType=sfix(16)  OutScaling=2^0
  Gain : Gain  Gain=Gain_Omega_r_m2  ParameterDataType=sfix(16)  ParameterScaling=2^0  OutDataType=sfix(16)  OutScaling=2^0
  Random Number : RandomNumber  Mean=m_omega_r  Variance=sigma_omega_r  Seed=seed(2)  SampleTime=Ts
  Random Number1 : RandomNumber  Mean=m_omega_r  Variance=sigma_omega_r  Seed=seed(3)  SampleTime=Ts
  Switch : Switch  Threshold=0.5
  Switch1 : Switch  Threshold=0.5
  Omega_r_m1 : Outport
  Omega_r_m2 : Outport  Port=2
  wires:
  Omega_r/1 -> Add/2, Add1/1
  Random Number/1 -> Add/1
  Random Number1/1 -> Add1/2
  Fault_4/1 -> Switch/2
  Constant/1 -> Switch/3
  Add/1 -> Switch/1
  Switch/1 -> Omega_r_m1/1
  Add1/1 -> Switch1/1, Gain/1
  Switch1/1 -> Omega_r_m2/1
  Fault_5/1 -> Switch1/2
  Gain/1 -> Switch1/3

== system FDIBenchMark_66/Sensors/P_g Sensor ==
  P_g : Inport
  Add : Sum  OutDataType=sfix(16)  OutScaling=2^-10
  Random Number : RandomNumber  Mean=m_P_g  Variance=sigma_P_g  Seed=seed(7)  SampleTime=Ts
  P_g_m : Outport
  wires:
  Random Number/1 -> Add/2
  P_g/1 -> Add/1
  Add/1 -> P_g_m/1

== system FDIBenchMark_66/Sensors/Pitch1 Sensor ==
  Beta_1 : Inport
  Fault_1 : Inport  Port=2
  Add : Sum  OutDataType=sfix(16)  OutScaling=2^-10
  Add1 : Sum  OutDataType=sfix(16)  OutScaling=2^-10
  Constant : Constant  Value=Constant_Beta_1_m1  OutDataType=sfix(16)  OutScaling=2^0
  Random Number : RandomNumber  Mean=m_Beta  Variance=sigma_Beta  Seed=seed(8)  SampleTime=Ts
  Random Number1 : RandomNumber  Mean=m_Beta  Variance=sigma_Beta  Seed=seed(9)  SampleTime=Ts
  Switch : Switch  Threshold=0.5
  Beta_1_m1 : Outport
  Beta_1_m2 : Outport  Port=2
  wires:
  Random Number1/1 -> Add1/2
  Add1/1 -> Beta_1_m2/1
  Random Number/1 -> Add/1
  Beta_1/1 -> Add1/1, Add/2
  Fault_1/1 -> Switch/2
  Constant/1 -> Switch/3
  Add/1 -> Switch/1
  Switch/1 -> Beta_1_m1/1

== system FDIBenchMark_66/Sensors/Pitch2 Sensor ==
  Beta_2 : Inport
  Fault_2 : Inport  Port=2
  Add : Sum  OutDataType=sfix(16)  OutScaling=2^-10
  Add1 : Sum  OutDataType=sfix(16)  OutScaling=2^-10
  Gain : Gain  Gain=Gain_Beta_2_m2  ParameterDataType=sfix(16)  ParameterScaling=2^0  OutDataType=sfix(16)  OutScaling=2^0
  Random Number : RandomNumber  Mean=m_Beta  Variance=sigma_Beta  Seed=seed(10)  SampleTime=Ts
  Random Number1 : RandomNumber  Mean=m_Beta  Variance=sigma_Beta  Seed=seed(11)  SampleTime=Ts
  Switch : Switch  Threshold=.5
  Beta_2_m1 : Outport
  Beta_2_m2 : Outport  Port=2
  wires:
  Random Number1/1 -> Add1/2
  Random Number/1 -> Add/1
  Beta_2/1 -> Add1/1, Add/2
  Add/1 -> Beta_2_m1/1
  Add1/1 -> Switch/1, Gain/1
  Gain/1 -> Switch/3
  Switch/1 -> Beta_2_m2/1
  Fault_2/1 -> Switch/2

== system FDIBenchMark_66/Sensors/Pitch3 Sensor ==
  Beta_3 : Inport
  Fault_3 : Inport  Port=2
  Add : Sum  OutDataType=sfix(16)  OutScaling=2^-10
  Add1 : Sum  OutDataType=sfix(16)  OutScaling=2^-10
  Constant : Constant  Value=Constant_Beta_3_m1  OutDataType=sfix(16)  OutScaling=2^0
  Random Number : RandomNumber  Mean=m_Beta  Variance=sigma_Beta  Seed=seed(12)  SampleTime=Ts
  Random Number1 : RandomNumber  Mean=m_Beta  Variance=sigma_Beta  Seed=seed(13)  SampleTime=Ts
  Switch : Switch  Threshold=0.5
  Beta_3_m1 : Outport
  Beta_3_m2 : Outport  Port=2
  wires:
  Random Number1/1 -> Add1/2
  Add1/1 -> Beta_3_m2/1
  Random Number/1 -> Add/1
  Beta_3/1 -> Add1/1, Add/2
  Fault_3/1 -> Switch/2
  Constant/1 -> Switch/3
  Add/1 -> Switch/1
  Switch/1 -> Beta_3_m1/1

== system FDIBenchMark_66/Sensors/Tau_g Sensor ==
  Tau_g : Inport
  Add : Sum  OutDataType=sfix(16)  OutScaling=2^-10
  Random Number : RandomNumber  Mean=m_tau_g  Variance=sigma_tau_g  Seed=seed(6)  SampleTime=Ts
  Tau_g_m : Outport
  wires:
  Add/1 -> Tau_g_m/1
  Tau_g/1 -> Add/1
  Random Number/1 -> Add/2

== system FDIBenchMark_66/Sensors/Wind Sensor ==
  v_hub : Inport
  Add : Sum  OutDataType=sfix(16)  OutScaling=2^-10
  Random Number : RandomNumber  Mean=m_vw  Variance=sigma_vm  Seed=seed(1)  SampleTime=Ts
  v_hub_m : Outport
  wires:
  Random Number/1 -> Add/2
  v_hub/1 -> Add/1
  Add/1 -> v_hub_m/1

== system FDIBenchMark_66/Wind model/3rd_Harmonic_Filter1 ==
  avg_wind : Inport  OutDataType=sfix(16)  OutScaling=2^0
  in_1 : Inport  Port=2  OutDataType=sfix(16)  OutScaling=2^0
  3rd harmonic Filter : Subsystem
  Unit Delay : UnitDelay  SampleTime=T_sample
  out_1 : Outport  OutDataType=sfix(16)  OutScaling=2^0
  wires:
  3rd harmonic Filter/1(Out) -> out_1/1
  avg_wind/1 -> 3rd harmonic Filter/1(avg_wind)
  in_1/1 -> Unit Delay/1
  Unit Delay/1 -> 3rd harmonic Filter/2(In)

== system FDIBenchMark_66/Wind model/Kaimal_Filter_1 ==
  in_1 : Inport  OutDataType=sfix(16)  OutScaling=2^0
  avg_wind : Inport  Port=2  OutDataType=sfix(16)  OutScaling=2^0
  Fcn : Fcn  Expr=turb_int*sqrt(L*u(1))/100/sqrt(2)
  Kaimal Filter : Subsystem
  Product : Product  OutDataType=sfix(16)  OutScaling=2^0  SaturateOnIntegerOverflow=on
  Unit Delay : UnitDelay  SampleTime=T_sample
  out_1 : Outport  OutDataType=sfix(16)  OutScaling=2^0
  wires:
  Product/1 -> out_1/1
  Kaimal Filter/1(Out) -> Product/2
  Fcn/1 -> Product/1
  avg_wind/1 -> Fcn/1, Kaimal Filter/1(avg_wind)
  in_1/1 -> Unit Delay/1
  Unit Delay/1 -> Kaimal Filter/2(In)

== system FDIBenchMark_66/Wind model/Kaimal_Filter_2 ==
  avg_wind : Inport  OutDataType=sfix(16)  OutScaling=2^0
  in_1 : Inport  Port=2  OutDataType=sfix(16)  OutScaling=2^0
  Fcn : Fcn  Expr=turb_int*sqrt(L*u(1))/100/sqrt(2)
  Kaimal Filter : Subsystem
  Product : Product  OutDataType=sfix(16)  OutScaling=2^0  SaturateOnIntegerOverflow=on
  Unit Delay : UnitDelay  SampleTime=T_sample
  out_1 : Outport  OutDataType=sfix(16)  OutScaling=2^0
  wires:
  Unit Delay/1 -> Kaimal Filter/2(In)
  in_1/1 -> Unit Delay/1
  avg_wind/1 -> Kaimal Filter/1(avg_wind), Fcn/1
  Fcn/1 -> Product/1
  Kaimal Filter/1(Out) -> Product/2
  Product/1 -> out_1/1

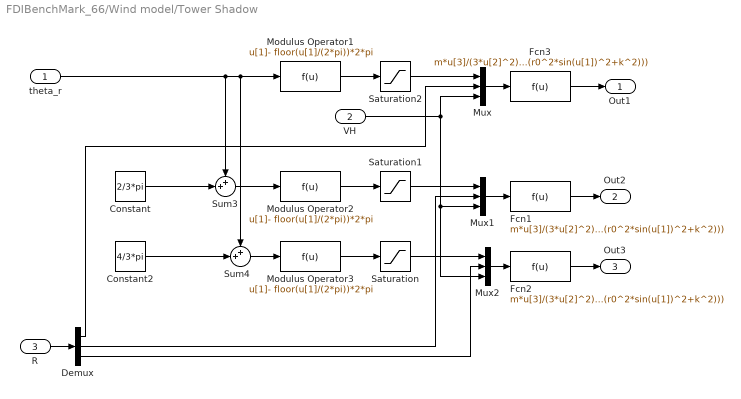
== system FDIBenchMark_66/Wind model/Tower Shadow ==
  theta_r : Inport  OutDataType=sfix(16)  OutScaling=2^0
  VH : Inport  Port=2  OutDataType=sfix(16)  OutScaling=2^0
  R : Inport  Port=3  OutDataType=sfix(16)  OutScaling=2^0
  Constant : Constant  Value=2/3*pi  OutDataType=sfix(16)  OutScaling=2^0
  Constant2 : Constant  Value=4/3*pi  OutDataType=sfix(16)  OutScaling=2^0
  Demux : Demux  Outputs=3
  Fcn1 : Fcn  Expr=m*u[3]/(3*u[2]^2)*(a^2*2*(u[2]^2-r0^2)/((u[2]^2+r0^2)*sin(u[1])^2+2*k^2)+2*a^2*k^2*(r0^2-u[2]^2)/((u[2]^2*sin(u[1])^2+k^2)*(r0^2*sin(u[1])^2+k^2)))
  Fcn2 : Fcn  Expr=m*u[3]/(3*u[2]^2)*(a^2*2*(u[2]^2-r0^2)/((u[2]^2+r0^2)*sin(u[1])^2+2*k^2)+2*a^2*k^2*(r0^2-u[2]^2)/((u[2]^2*sin(u[1])^2+k^2)*(r0^2*sin(u[1])^2+k^2)))
  Fcn3 : Fcn  Expr=m*u[3]/(3*u[2]^2)*(a^2*2*(u[2]^2-r0^2)/((u[2]^2+r0^2)*sin(u[1])^2+2*k^2)+2*a^2*k^2*(r0^2-u[2]^2)/((u[2]^2*sin(u[1])^2+k^2)*(r0^2*sin(u[1])^2+k^2)))
  Modulus Operator1 : Fcn  Expr=u[1]- floor(u[1]/(2*pi))*2*pi
  Modulus Operator2 : Fcn  Expr=u[1]- floor(u[1]/(2*pi))*2*pi
  Modulus Operator3 : Fcn  Expr=u[1]- floor(u[1]/(2*pi))*2*pi
  Mux : Mux  Inputs=3
  Mux1 : Mux  Inputs=3
  Mux2 : Mux  Inputs=3
  Saturation : Saturate  UpperLimit=3*pi/2  LowerLimit=pi/2
  Saturation1 : Saturate  UpperLimit=3*pi/2  LowerLimit=pi/2
  Saturation2 : Saturate  UpperLimit=3*pi/2  LowerLimit=pi/2
  Sum3 : Sum  Inputs=++|  OutDataType=sfix(16)  OutScaling=2^0
  Sum4 : Sum  Inputs=++|  OutDataType=sfix(16)  OutScaling=2^0
  Out1 : Outport
  Out2 : Outport  Port=2
  Out3 : Outport  Port=3
  wires:
  theta_r/1 -> Sum3/1, Sum4/1, Modulus Operator1/1
  Sum4/1 -> Modulus Operator3/1
  Constant2/1 -> Sum4/2
  Sum3/1 -> Modulus Operator2/1
  Constant/1 -> Sum3/2
  Modulus Operator1/1 -> Saturation2/1
  Modulus Operator2/1 -> Saturation1/1
  Modulus Operator3/1 -> Saturation/1
  Mux/1 -> Fcn3/1
  Saturation2/1 -> Mux/1
  Demux/1 -> Mux/2
  R/1 -> Demux/1
  Mux1/1 -> Fcn1/1
  Saturation1/1 -> Mux1/1
  Demux/2 -> Mux1/2
  Mux2/1 -> Fcn2/1
  Saturation/1 -> Mux2/1
  Demux/3 -> Mux2/2
  VH/1 -> Mux/3, Mux2/3, Mux1/3
  Fcn3/1 -> Out1/1
  Fcn1/1 -> Out2/1
  Fcn2/1 -> Out3/1

== system FDIBenchMark_66/Wind model/White Noise_1 ==
  Gain : Gain  Gain=[sqrt(Cov)]/[sqrt(Ts)]  ParameterDataType=sfix(16)  ParameterScaling=2^0  OutDataType=sfix(16)  OutScaling=2^0  SaturateOnIntegerOverflow=on
  White Noise : RandomNumber  Seed=seed  SampleTime=Ts
  Zero-Order Hold : ZeroOrderHold  SampleTime=Ts
  Out_1 : Outport  OutDataType=sfix(16)  OutScaling=2^0
  wires:
  White Noise/1 -> Zero-Order Hold/1
  Gain/1 -> Out_1/1
  Zero-Order Hold/1 -> Gain/1

== system FDIBenchMark_66/Wind model/White Noise_2 ==
  Gain : Gain  Gain=[sqrt(Cov)]/[sqrt(Ts)]  ParameterDataType=sfix(16)  ParameterScaling=2^0  OutDataType=sfix(16)  OutScaling=2^0  SaturateOnIntegerOverflow=on
  White Noise : RandomNumber  Seed=seed  SampleTime=Ts
  Zero-Order Hold : ZeroOrderHold  SampleTime=Ts
  Out_1 : Outport  OutDataType=sfix(16)  OutScaling=2^0
  wires:
  White Noise/1 -> Zero-Order Hold/1
  Gain/1 -> Out_1/1
  Zero-Order Hold/1 -> Gain/1

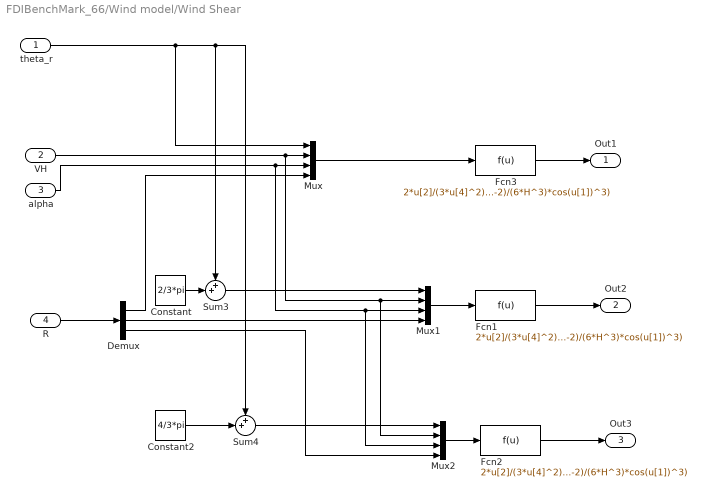
== system FDIBenchMark_66/Wind model/Wind Shear ==
  theta_r : Inport  OutDataType=sfix(16)  OutScaling=2^0
  VH : Inport  Port=2  OutDataType=sfix(16)  OutScaling=2^0
  alpha : Inport  Port=3  OutDataType=sfix(16)  OutScaling=2^0
  R : Inport  Port=4  OutDataType=sfix(16)  OutScaling=2^0
  Constant : Constant  Value=2/3*pi  OutDataType=sfix(16)  OutScaling=2^0
  Constant2 : Constant  Value=4/3*pi  OutDataType=sfix(16)  OutScaling=2^0
  Demux : Demux  Outputs=3
  Fcn1 : Fcn  Expr=2*u[2]/(3*u[4]^2)*(u[4]^3/3*u[3]/H*cos(u[1])+u[4]^4/4*u[3]*(u[3]-1)/(2*H^2)*cos(u[1])^2+u[4]^5/5*u[3]*(u[3]-1)*(u[3]-2)/(6*H^3)*cos(u[1])^3)
  Fcn2 : Fcn  Expr=2*u[2]/(3*u[4]^2)*(u[4]^3/3*u[3]/H*cos(u[1])+u[4]^4/4*u[3]*(u[3]-1)/(2*H^2)*cos(u[1])^2+u[4]^5/5*u[3]*(u[3]-1)*(u[3]-2)/(6*H^3)*cos(u[1])^3)
  Fcn3 : Fcn  Expr=2*u[2]/(3*u[4]^2)*(u[4]^3/3*u[3]/H*cos(u[1])+u[4]^4/4*u[3]*(u[3]-1)/(2*H^2)*cos(u[1])^2+u[4]^5/5*u[3]*(u[3]-1)*(u[3]-2)/(6*H^3)*cos(u[1])^3)
  Mux : Mux
  Mux1 : Mux
  Mux2 : Mux
  Sum3 : Sum  Inputs=++|  OutDataType=sfix(16)  OutScaling=2^0
  Sum4 : Sum  Inputs=++|  OutDataType=sfix(16)  OutScaling=2^0
  Out1 : Outport
  Out2 : Outport  Port=2
  Out3 : Outport  Port=3
  wires:
  theta_r/1 -> Sum3/1, Sum4/1, Mux/1
  VH/1 -> Mux/2, Mux1/2, Mux2/2
  Sum4/1 -> Mux2/1
  Constant2/1 -> Sum4/2
  Sum3/1 -> Mux1/1
  Constant/1 -> Sum3/2
  alpha/1 -> Mux/3, Mux1/3, Mux2/3
  Fcn2/1 -> Out3/1
  Fcn1/1 -> Out2/1
  Mux/1 -> Fcn3/1
  R/1 -> Demux/1
  Demux/1 -> Mux/4
  Mux1/1 -> Fcn1/1
  Mux2/1 -> Fcn2/1
  Demux/2 -> Mux1/4
  Demux/3 -> Mux2/4
  Fcn3/1 -> Out1/1

== system FDIBenchMark_66/Wind model/ZERO_Harmonic_Filter ==
  in_1 : Inport  OutDataType=sfix(16)  OutScaling=2^0
  avg_wind : Inport  Port=2  OutDataType=sfix(16)  OutScaling=2^0
  Unit Delay : UnitDelay  SampleTime=T_sample
  ZERO harmonic Filter : Subsystem
  out_1 : Outport  OutDataType=sfix(16)  OutScaling=2^0
  wires:
  Unit Delay/1 -> ZERO harmonic Filter/2(In)
  in_1/1 -> Unit Delay/1
  avg_wind/1 -> ZERO harmonic Filter/1(avg_wind)
  ZERO harmonic Filter/1(Out) -> out_1/1

== system FDIBenchMark_66/Blade&Pitch System/Pitch Systems/PitchSystem 1 ==
  Beta_r : Inport  OutDataType=sfix(16)  OutScaling=2^0
  Transfer Fcn : TransferFcn  Numerator=[omega_n^2]  Denominator=[1 2*xi*omega_n omega_n^2]
  Beta_1 : Outport  OutDataType=sfix(16)  OutScaling=2^0
  wires:
  Beta_r/1 -> Transfer Fcn/1
  Transfer Fcn/1 -> Beta_1/1

== system FDIBenchMark_66/Blade&Pitch System/Pitch Systems/PitchSystem 2 ==
  Beta_r : Inport  OutDataType=sfix(16)  OutScaling=2^0
  Fault_6 : Inport  Port=2  OutDataType=sfix(16)  OutScaling=2^0
  Add : Sum  OutDataType=sfix(16)  OutScaling=2^-10
  Gain : Gain  Orientation=left  Gain=Apb  Multiplication=Matrix(K*u)  ParameterDataType=sfix(16)  ParameterScaling=2^0  OutDataType=sfix(16)  OutScaling=2^0
  Gain1 : Gain  Gain=Bpb  Multiplication=Matrix(K*u)  ParameterDataType=sfix(16)  ParameterScaling=2^0  OutDataType=sfix(16)  OutScaling=2^0
  Gain2 : Gain  Gain=Cpb  Multiplication=Matrix(K*u)  ParameterDataType=sfix(16)  ParameterScaling=2^0  OutDataType=sfix(16)  OutScaling=2^0
  Gain3 : Gain  Orientation=left  Gain=Apb1  Multiplication=Matrix(K*u)  ParameterDataType=sfix(16)  ParameterScaling=2^0  OutDataType=sfix(16)  OutScaling=2^0
  Gain4 : Gain  Gain=Bpb1  Multiplication=Matrix(K*u)  ParameterDataType=sfix(16)  ParameterScaling=2^0  OutDataType=sfix(16)  OutScaling=2^0
  Gain5 : Gain  Gain=Cpb1  Multiplication=Matrix(K*u)  ParameterDataType=sfix(16)  ParameterScaling=2^0  OutDataType=sfix(16)  OutScaling=2^0
  Integrator : Integrator
  Switch1 : Switch  Threshold=0.5
  Switch2 : Switch  Orientation=left  Threshold=0.5
  Switch3 : Switch  Threshold=0.5
  Beta_2 : Outport  OutDataType=sfix(16)  OutScaling=2^0
  wires:
  Integrator/1 -> Gain/1, Gain3/1, Gain2/1, Gain5/1
  Add/1 -> Integrator/1
  Switch1/1 -> Add/1
  Gain1/1 -> Switch1/1
  Gain4/1 -> Switch1/3
  Gain/1 -> Switch2/1
  Gain3/1 -> Switch2/3
  Switch2/1 -> Add/2
  Fault_6/1 -> Switch1/2, Switch2/2, Switch3/2
  Beta_r/1 -> Gain1/1, Gain4/1
  Gain2/1 -> Switch3/1
  Switch3/1 -> Beta_2/1
  Gain5/1 -> Switch3/3

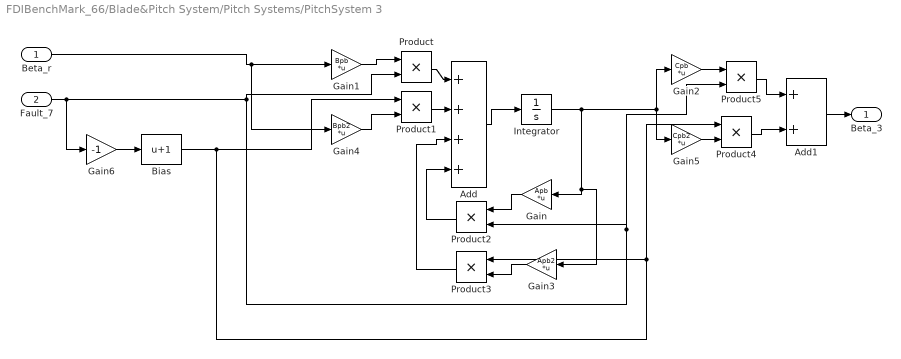
== system FDIBenchMark_66/Blade&Pitch System/Pitch Systems/PitchSystem 3 ==
  Beta_r : Inport  OutDataType=sfix(16)  OutScaling=2^0
  Fault_7 : Inport  Port=2  OutDataType=sfix(16)  OutScaling=2^0
  Add : Sum  Inputs=++++  OutDataType=sfix(16)  OutScaling=2^-10
  Add1 : Sum  OutDataType=sfix(16)  OutScaling=2^-10
  Bias : Bias  Bias=1
  Gain : Gain  Orientation=left  Gain=Apb  Multiplication=Matrix(K*u)  ParameterDataType=sfix(16)  ParameterScaling=2^0  OutDataType=sfix(16)  OutScaling=2^0
  Gain1 : Gain  Gain=Bpb  Multiplication=Matrix(K*u)  ParameterDataType=sfix(16)  ParameterScaling=2^0  OutDataType=sfix(16)  OutScaling=2^0
  Gain2 : Gain  Gain=Cpb  Multiplication=Matrix(K*u)  ParameterDataType=sfix(16)  ParameterScaling=2^0  OutDataType=sfix(16)  OutScaling=2^0
  Gain3 : Gain  Orientation=left  Gain=Apb2  Multiplication=Matrix(K*u)  ParameterDataType=sfix(16)  ParameterScaling=2^0  OutDataType=sfix(16)  OutScaling=2^0
  Gain4 : Gain  Gain=Bpb2  Multiplication=Matrix(K*u)  ParameterDataType=sfix(16)  ParameterScaling=2^0  OutDataType=sfix(16)  OutScaling=2^0
  Gain5 : Gain  Gain=Cpb2  Multiplication=Matrix(K*u)  ParameterDataType=sfix(16)  ParameterScaling=2^0  OutDataType=sfix(16)  OutScaling=2^0
  Gain6 : Gain  Gain=-1  ParameterDataType=sfix(16)  ParameterScaling=2^0  OutDataType=sfix(16)  OutScaling=2^0
  Integrator : Integrator
  Product{,1,4..5} (4 alike) : Product  OutDataType=sfix(16)  OutScaling=2^0  RndMeth=Zero
  Product2 : Product  Orientation=left  OutDataType=sfix(16)  OutScaling=2^0  RndMeth=Zero
  Product3 : Product  Orientation=left  OutDataType=sfix(16)  OutScaling=2^0  RndMeth=Zero
  Beta_3 : Outport  OutDataType=sfix(16)  OutScaling=2^0
  wires:
  Beta_r/1 -> Gain4/1, Gain1/1
  Fault_7/1 -> Product2/2, Product5/2, Product/2, Gain6/1
  Gain4/1 -> Product1/2
  Add/1 -> Integrator/1
  Integrator/1 -> Gain5/1, Gain2/1, Gain3/1, Gain/1
  Product/1 -> Add/1
  Gain1/1 -> Product/1
  Product1/1 -> Add/2
  Gain3/1 -> Product3/2
  Gain/1 -> Product2/1
  Product2/1 -> Add/4
  Product3/1 -> Add/3
  Add1/1 -> Beta_3/1
  Gain2/1 -> Product5/1
  Gain5/1 -> Product4/2
  Product4/1 -> Add1/2
  Product5/1 -> Add1/1
  Gain6/1 -> Bias/1
  Bias/1 -> Product1/1, Product3/1, Product4/1

== system FDIBenchMark_66/Blade&Pitch System/Subsystem/AeroDyn 1 ==
  v_w : Inport  Orientation=down
  Omega_r : Inport  Port=2
  Beta_1 : Inport  Port=3
  Divide : Product  Inputs=/*  OutDataType=sfix(16)  OutScaling=2^-10
  Divide1 : Product  Inputs=***  OutDataType=sfix(16)  OutScaling=2^-10
  Gain : Gain  Gain=R  ParameterDataType=sfix(16)  ParameterScaling=2^0  OutDataType=sfix(16)  OutScaling=2^0
  Gain1 : Gain  Gain=rho*pi*R^3/6  ParameterDataType=sfix(16)  ParameterScaling=2^0  OutDataType=sfix(16)  OutScaling=2^0
  Lookup Table (2-D) : Lookup2D  RowIndex=Lambda  ColumnIndex=Angle  OutputValues=Cq  OutDataType=sfix(16)  OutScaling=2^0
  Tau_r1 : Outport
  wires:
  Divide/1 -> Lookup Table (2-D)/1
  Gain/1 -> Divide/2
  v_w/1 -> Divide/1, Divide1/2, Divide1/1
  Lookup Table (2-D)/1 -> Divide1/3
  Divide1/1 -> Gain1/1
  Omega_r/1 -> Gain/1
  Gain1/1 -> Tau_r1/1
  Beta_1/1 -> Lookup Table (2-D)/2

== system FDIBenchMark_66/Blade&Pitch System/Subsystem/AeroDyn 2 ==
  v_w : Inport  Orientation=down
  Omega_r : Inport  Port=2
  Beta_2 : Inport  Port=3
  Divide : Product  Inputs=/*  OutDataType=sfix(16)  OutScaling=2^-10
  Divide1 : Product  Inputs=***  OutDataType=sfix(16)  OutScaling=2^-10
  Gain : Gain  Gain=R  ParameterDataType=sfix(16)  ParameterScaling=2^0  OutDataType=sfix(16)  OutScaling=2^0
  Gain1 : Gain  Gain=rho*pi*R^3/6  ParameterDataType=sfix(16)  ParameterScaling=2^0  OutDataType=sfix(16)  OutScaling=2^0
  Lookup Table (2-D) : Lookup2D  RowIndex=Lambda  ColumnIndex=Angle  OutputValues=Cq  OutDataType=sfix(16)  OutScaling=2^0
  Tau_r2 : Outport
  wires:
  Beta_2/1 -> Lookup Table (2-D)/2
  Gain1/1 -> Tau_r2/1
  Omega_r/1 -> Gain/1
  Divide1/1 -> Gain1/1
  Lookup Table (2-D)/1 -> Divide1/3
  v_w/1 -> Divide1/1, Divide1/2, Divide/1
  Gain/1 -> Divide/2
  Divide/1 -> Lookup Table (2-D)/1

== system FDIBenchMark_66/Blade&Pitch System/Subsystem/AeroDyn 3 ==
  v_w : Inport  Orientation=down
  Omega_r : Inport  Port=2
  Beta_3 : Inport  Port=3
  Divide : Product  Inputs=/*  OutDataType=sfix(16)  OutScaling=2^-10
  Divide1 : Product  Inputs=***  OutDataType=sfix(16)  OutScaling=2^-10
  Gain : Gain  Gain=R  ParameterDataType=sfix(16)  ParameterScaling=2^0  OutDataType=sfix(16)  OutScaling=2^0
  Gain1 : Gain  Gain=rho*pi*R^3/6  ParameterDataType=sfix(16)  ParameterScaling=2^0  OutDataType=sfix(16)  OutScaling=2^0
  Lookup Table (2-D) : Lookup2D  RowIndex=Lambda  ColumnIndex=Angle  OutputValues=Cq  OutDataType=sfix(16)  OutScaling=2^0
  Tau_r3 : Outport
  wires:
  Divide/1 -> Lookup Table (2-D)/1
  Gain/1 -> Divide/2
  v_w/1 -> Divide/1, Divide1/2, Divide1/1
  Lookup Table (2-D)/1 -> Divide1/3
  Divide1/1 -> Gain1/1
  Omega_r/1 -> Gain/1
  Gain1/1 -> Tau_r3/1
  Beta_3/1 -> Lookup Table (2-D)/2

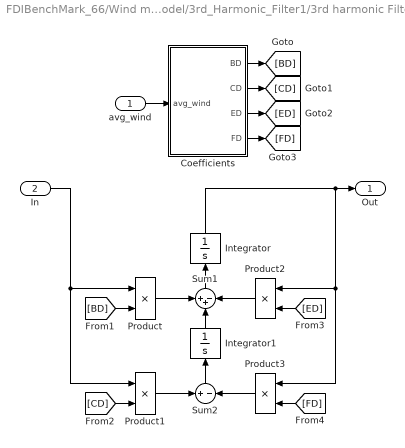
== system FDIBenchMark_66/Wind model/3rd_Harmonic_Filter1/3rd harmonic Filter ==
  avg_wind : Inport  OutDataType=sfix(16)  OutScaling=2^0
  In : Inport  Port=2  OutDataType=sfix(16)  OutScaling=2^0
  Coefficients : Subsystem
  Integrator : Integrator  Orientation=up
  Integrator1 : Integrator  Orientation=up
  Product : Product  OutDataType=sfix(16)  OutScaling=2^0  SaturateOnIntegerOverflow=on
  Product1 : Product  OutDataType=sfix(16)  OutScaling=2^0  SaturateOnIntegerOverflow=on
  Product2 : Product  Orientation=left  OutDataType=sfix(16)  OutScaling=2^0  SaturateOnIntegerOverflow=on
  Product3 : Product  Orientation=left  OutDataType=sfix(16)  OutScaling=2^0  SaturateOnIntegerOverflow=on
  Sum1 : Sum  Orientation=up  Inputs=++-  OutDataType=sfix(16)  OutScaling=2^0  SaturateOnIntegerOverflow=on
  Sum2 : Sum  Orientation=up  Inputs=+|-  OutDataType=sfix(16)  OutScaling=2^0  SaturateOnIntegerOverflow=on
  Out : Outport  OutDataType=sfix(16)  OutScaling=2^0
  wires:
  avg_wind/1 -> Coefficients/1(avg_wind)
  Coefficients/4(FD) -> [FD]
  Coefficients/3(ED) -> [ED]
  Coefficients/2(CD) -> [CD]
  Coefficients/1(BD) -> [BD]
  [FD] -> Product3/2
  [ED] -> Product2/2
  [CD] -> Product1/2
  [BD] -> Product/2
  In/1 -> Product1/1, Product/1
  Product1/1 -> Sum2/1
  Product3/1 -> Sum2/2
  Sum2/1 -> Integrator1/1
  Product2/1 -> Sum1/3
  Integrator1/1 -> Sum1/2
  Product/1 -> Sum1/1
  Sum1/1 -> Integrator/1
  Integrator/1 -> Out/1, Product3/1, Product2/1

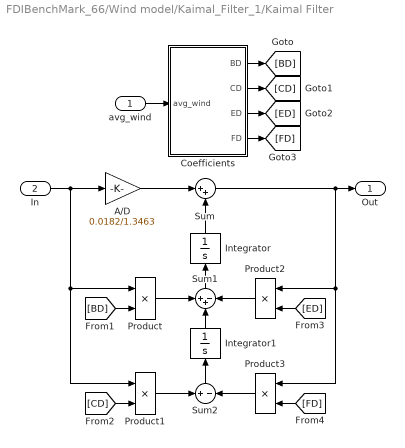
== system FDIBenchMark_66/Wind model/Kaimal_Filter_1/Kaimal Filter ==
  avg_wind : Inport  OutDataType=sfix(16)  OutScaling=2^0
  In : Inport  Port=2  OutDataType=sfix(16)  OutScaling=2^0
  A/D : Gain  Gain=0.0182/1.3463  ParameterDataType=sfix(16)  ParameterScaling=2^0  OutDataType=sfix(16)  OutScaling=2^0  SaturateOnIntegerOverflow=on
  Coefficients : Subsystem
  Integrator : Integrator  Orientation=up
  Integrator1 : Integrator  Orientation=up
  Product : Product  OutDataType=sfix(16)  OutScaling=2^0  SaturateOnIntegerOverflow=on
  Product1 : Product  OutDataType=sfix(16)  OutScaling=2^0  SaturateOnIntegerOverflow=on
  Product2 : Product  Orientation=left  OutDataType=sfix(16)  OutScaling=2^0  SaturateOnIntegerOverflow=on
  Product3 : Product  Orientation=left  OutDataType=sfix(16)  OutScaling=2^0  SaturateOnIntegerOverflow=on
  Sum : Sum  Inputs=|++  OutDataType=sfix(16)  OutScaling=2^0  SaturateOnIntegerOverflow=on
  Sum1 : Sum  Orientation=up  Inputs=++-  OutDataType=sfix(16)  OutScaling=2^0  SaturateOnIntegerOverflow=on
  Sum2 : Sum  Orientation=up  Inputs=+|-  OutDataType=sfix(16)  OutScaling=2^0  SaturateOnIntegerOverflow=on
  Out : Outport  OutDataType=sfix(16)  OutScaling=2^0
  wires:
  avg_wind/1 -> Coefficients/1(avg_wind)
  Coefficients/4(FD) -> [FD]
  Coefficients/3(ED) -> [ED]
  Coefficients/2(CD) -> [CD]
  Coefficients/1(BD) -> [BD]
  [FD] -> Product3/2
  [ED] -> Product2/2
  [CD] -> Product1/2
  [BD] -> Product/2
  In/1 -> Product1/1, Product/1, A/D/1
  Sum/1 -> Out/1, Product3/1, Product2/1
  Product1/1 -> Sum2/1
  Product3/1 -> Sum2/2
  Sum2/1 -> Integrator1/1
  Product2/1 -> Sum1/3
  Integrator1/1 -> Sum1/2
  Product/1 -> Sum1/1
  Sum1/1 -> Integrator/1
  Integrator/1 -> Sum/2
  A/D/1 -> Sum/1
